simulink model "projeto3a"  (Simulink 5.0)
settings: Solver=ode45  StartTime=0.0  StopTime=10  RelTol=1e-3
settings Model: LastModifiedBy=Frank Gloria

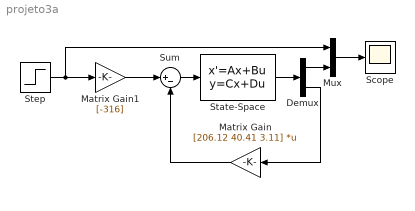
== system projeto3a ==
  Demux : Demux  Outputs=2
  Matrix Gain : Gain  Orientation=left  Gain=[206.12 40.41 3.11]  Multiplication=Matrix(K*u) (u vector)  SaturateOnIntegerOverflow=on
  Matrix Gain1 : Gain  Gain=[-316]  SaturateOnIntegerOverflow=on
  Mux : Mux  Inputs=2
  Scope : Scope
  State-Space : StateSpace  A=[1 1 0; -1.5 0 1;137.5 0 0]  B=[0;1;2]  C=[1 2 0; 1 0 0;0 1 0; 0 0 1]  D=[0; 0; 0; 0]
  Step : Step  Time=0  SampleTime=0
  Sum : Sum  Inputs=|+-  SaturateOnIntegerOverflow=on
  wires:
  Demux/2 -> Matrix Gain/1
  Step/1 -> Mux/1, Matrix Gain1/1
  State-Space/1 -> Demux/1
  Matrix Gain/1 -> Sum/2
  Sum/1 -> State-Space/1
  Demux/1 -> Mux/2
  Mux/1 -> Scope/1
  Matrix Gain1/1 -> Sum/1
